simulink model "model"  (Simulink 7.9)
settings: Solver=ode3  StartTime=0.0  StopTime=5  FixedStep=0.001  RelTol=1e-3
values from neighbouring files (symbols this model uses):
  a = -1.0    (= -1)    [parameters.m]
  Ah = 0.234    [parameters.m]
  Ak = 0.227    [parameters.m]
  b = -2.0    (= -2)    [parameters.m]
  c = 0.23    [parameters.m]
  p = 0.1786    [parameters.m]
  Ta = 0.38    [parameters.m]
  Tr = 0.04    [parameters.m]
  U0 = 0.1*rand(4,4)    [parameters.m]
  W = [0 -1 1 -1; -1 0 -1 1; 1 -1 0 -1; -1 1 -1 0]    [parameters.m]
settings Model: Creator=dede  LastModifiedBy=dede

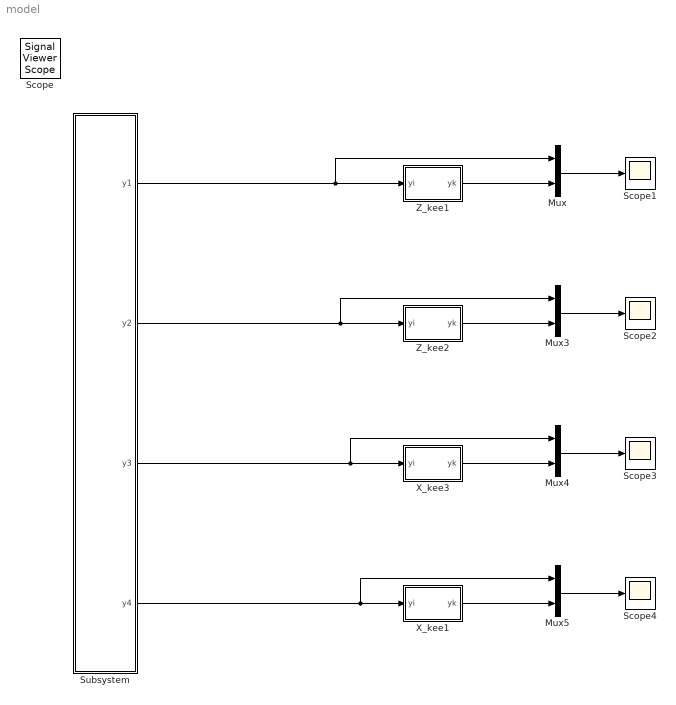
== system model ==
  Mux{,3..5} (4 alike) : Mux  Inputs=2
  Scope{1..4} (4 alike) : Scope
      Scope3 settings: SaveName=ScopeData2
      Scope4 settings: SaveName=ScopeData3
  Subsystem : Subsystem
  X_kee1 : Subsystem
  X_kee3 : Subsystem
  Z_kee1 : Subsystem
  Z_kee2 : Subsystem
  Scope : SignalViewerScope  IOType=viewer  NumInputPorts=4  RefreshTime=0.035000
      settings: YMin=-5~-5~-5~-5  YMax=5~5~5~5
  wires:
  Z_kee1/1(yk) -> Mux/2
  Mux/1 -> Scope1/1
  Z_kee2/1(yk) -> Mux3/2
  Mux3/1 -> Scope2/1
  X_kee3/1(yk) -> Mux4/2
  Mux4/1 -> Scope3/1
  Mux5/1 -> Scope4/1
  X_kee1/1(yk) -> Mux5/2
  Subsystem/4(y4) -> X_kee1/1(yi), Mux5/1
  Subsystem/3(y3) -> X_kee3/1(yi), Mux4/1
  Subsystem/2(y2) -> Z_kee2/1(yi), Mux3/1
  Subsystem/1(y1) -> Z_kee1/1(yi), Mux/1

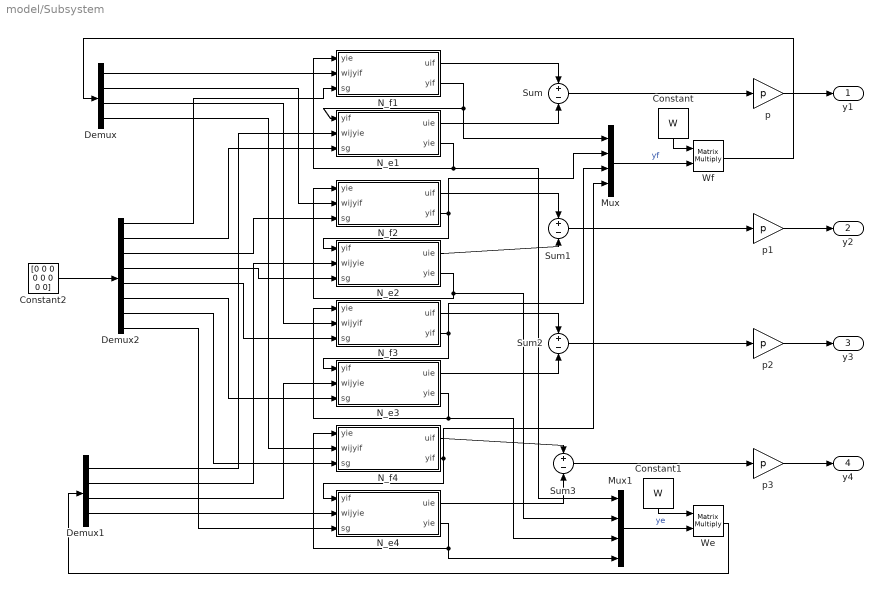
== system model/Subsystem ==
  Constant : Constant  Value=W
  Constant1 : Constant  Value=W
  Constant2 : Constant  Value=[0 0 0 0 0 0 0 0]
  Demux : Demux
  Demux1 : Demux
  Demux2 : Demux  Outputs=8
  Mux : Mux
  Mux1 : Mux
  N_e1 : Subsystem
  N_e2 : Subsystem
  N_e3 : Subsystem
  N_e4 : Subsystem
  N_f1 : Subsystem
  N_f2 : Subsystem
  N_f3 : Subsystem
  N_f4 : Subsystem
  Sum{,1..3} (4 alike) : Sum  Inputs=+-
  We : Product  Multiplication=Matrix(*)  RndMeth=Zero
  Wf : Product  Multiplication=Matrix(*)  RndMeth=Zero
  p{,1..3} (4 alike) : Gain  Gain=p
  y1 : Outport
  y2 : Outport  Port=2
  y3 : Outport  Port=3
  y4 : Outport  Port=4
  wires:
  N_f1/2(yif) -> N_e1/1(yif), Mux/1
  N_e1/2(yie) -> N_f1/1(yie), Mux1/1
  N_f2/2(yif) -> N_e2/1(yif), Mux/2
  N_e2/2(yie) -> N_f2/1(yie), Mux1/2
  N_f3/2(yif) -> N_e3/1(yif), Mux/3
  N_e3/2(yie) -> N_f3/1(yie), Mux1/3
  N_f4/2(yif) -> N_e4/1(yif), Mux/4
  N_e4/2(yie) -> N_f4/1(yie), Mux1/4
  N_f1/1(uif) -> Sum/1
  N_e1/1(uie) -> Sum/2
  N_f2/1(uif) -> Sum1/1
  N_e2/1(uie) -> Sum1/2
  N_f3/1(uif) -> Sum2/1
  N_e3/1(uie) -> Sum2/2
  N_f4/1(uif) -> Sum3/1
  N_e4/1(uie) -> Sum3/2
  Sum/1 -> p/1
  Mux/1 -> Wf/2  "yf"
  Constant/1 -> Wf/1
  Wf/1 -> Demux/1
  Mux1/1 -> We/2  "ye"
  Constant1/1 -> We/1
  We/1 -> Demux1/1
  Demux/1 -> N_f1/2(wijyif)
  Demux/2 -> N_f2/2(wijyif)
  Demux/3 -> N_f3/2(wijyif)
  Demux/4 -> N_f4/2(wijyif)
  Demux1/1 -> N_e1/2(wijyie)
  Demux1/2 -> N_e2/2(wijyie)
  Demux1/3 -> N_e3/2(wijyie)
  Demux1/4 -> N_e4/2(wijyie)
  Constant2/1 -> Demux2/1
  Demux2/1 -> N_f1/3(sg)
  Demux2/2 -> N_e1/3(sg)
  Demux2/3 -> N_f2/3(sg)
  Demux2/4 -> N_e2/3(sg)
  Demux2/5 -> N_f3/3(sg)
  Demux2/6 -> N_e3/3(sg)
  Demux2/7 -> N_f4/3(sg)
  Demux2/8 -> N_e4/3(sg)
  Sum1/1 -> p1/1
  p1/1 -> y2/1
  Sum2/1 -> p2/1
  p2/1 -> y3/1
  Sum3/1 -> p3/1
  p3/1 -> y4/1
  p/1 -> y1/1

== system model/X_kee1 ==
  yi : Inport
  Constant2 : Constant  Value=0
  Derivative : Derivative
  Subsystem : Subsystem
  Switch : Switch
  yk : Outport
  wires:
  Switch/1 -> yk/1
  Subsystem/1(Out1) -> Switch/1
  Derivative/1 -> Switch/2
  yi/1 -> Subsystem/1(In1), Derivative/1
  Constant2/1 -> Switch/3

== system model/X_kee3 ==
  yi : Inport
  Constant2 : Constant  Value=0
  Derivative : Derivative
  Subsystem : Subsystem
  Switch : Switch
  yk : Outport
  wires:
  Constant2/1 -> Switch/3
  yi/1 -> Derivative/1, Subsystem/1(In1)
  Derivative/1 -> Switch/2
  Subsystem/1(Out1) -> Switch/1
  Switch/1 -> yk/1

== system model/Z_kee1 ==
  yi : Inport
  Constant2 : Constant  Value=0
  Derivative : Derivative
  Subsystem : Subsystem
  Switch : Switch
  yk : Outport
  wires:
  Constant2/1 -> Switch/3
  yi/1 -> Derivative/1, Subsystem/1(In1)
  Derivative/1 -> Switch/2
  Subsystem/1(Out1) -> Switch/1
  Switch/1 -> yk/1

== system model/Z_kee2 ==
  yi : Inport
  Constant2 : Constant  Value=0
  Derivative : Derivative
  Subsystem : Subsystem
  Switch : Switch
  yk : Outport
  wires:
  Switch/1 -> yk/1
  Subsystem/1(Out1) -> Switch/1
  Derivative/1 -> Switch/2
  yi/1 -> Subsystem/1(In1), Derivative/1
  Constant2/1 -> Switch/3

== system model/Subsystem/N_e1 ==
  yif : Inport
  wijyie : Inport  Port=2
  sg : Inport  Port=3
  Constant : Constant  Value=0
  uie0 : Subsystem
  vie : Subsystem
  yie0 : Switch
  uie : Outport
  yie : Outport  Port=2
  wires:
  vie/1(vie) -> uie0/1(vie)
  yif/1 -> uie0/2(yif)
  wijyie/1 -> uie0/3(wijyie)
  Constant/1 -> yie0/3
  uie0/1(uie) -> yie0/1, yie0/2, uie/1
  yie0/1 -> vie/1(yie), yie/1
  sg/1 -> uie0/4(sg)

== system model/Subsystem/N_e2 ==
  yif : Inport
  wijyie : Inport  Port=2
  sg : Inport  Port=3
  Constant : Constant  Value=0
  uie0 : Subsystem
  vie : Subsystem
  yie0 : Switch
  uie : Outport
  yie : Outport  Port=2
  wires:
  sg/1 -> uie0/4(sg)
  yie0/1 -> yie/1, vie/1(yie)
  uie0/1(uie) -> uie/1, yie0/2, yie0/1
  Constant/1 -> yie0/3
  wijyie/1 -> uie0/3(wijyie)
  yif/1 -> uie0/2(yif)
  vie/1(vie) -> uie0/1(vie)

== system model/Subsystem/N_e3 ==
  yif : Inport
  wijyie : Inport  Port=2
  sg : Inport  Port=3
  Constant : Constant  Value=0
  uie0 : Subsystem
  vie : Subsystem
  yie0 : Switch
  uie : Outport
  yie : Outport  Port=2
  wires:
  vie/1(vie) -> uie0/1(vie)
  yif/1 -> uie0/2(yif)
  wijyie/1 -> uie0/3(wijyie)
  Constant/1 -> yie0/3
  uie0/1(uie) -> yie0/1, yie0/2, uie/1
  yie0/1 -> vie/1(yie), yie/1
  sg/1 -> uie0/4(sg)

== system model/Subsystem/N_e4 ==
  yif : Inport
  wijyie : Inport  Port=2
  sg : Inport  Port=3
  Constant : Constant  Value=0
  uie0 : Subsystem
  vie : Subsystem
  yie0 : Switch
  uie : Outport
  yie : Outport  Port=2
  wires:
  sg/1 -> uie0/4(sg)
  yie0/1 -> yie/1, vie/1(yie)
  uie0/1(uie) -> uie/1, yie0/2, yie0/1
  Constant/1 -> yie0/3
  wijyie/1 -> uie0/3(wijyie)
  yif/1 -> uie0/2(yif)
  vie/1(vie) -> uie0/1(vie)

== system model/Subsystem/N_f1 ==
  yie : Inport
  wijyif : Inport  Port=2
  sg : Inport  Port=3
  Constant : Constant  Value=0
  uif0 : Subsystem
  vif : Subsystem
  yif0 : Switch
  uif : Outport
  yif : Outport  Port=2
  wires:
  vif/1(vif) -> uif0/1(vif)
  Constant/1 -> yif0/3
  uif0/1(uif) -> yif0/1, yif0/2, uif/1
  yif0/1 -> yif/1, vif/1(yif)
  yie/1 -> uif0/2(yie)
  wijyif/1 -> uif0/3(wijyif)
  sg/1 -> uif0/4(sg)

== system model/Subsystem/N_f2 ==
  yie : Inport
  wijyif : Inport  Port=2
  sg : Inport  Port=3
  Constant : Constant  Value=0
  uif0 : Subsystem
  vif : Subsystem
  yif0 : Switch
  uif : Outport
  yif : Outport  Port=2
  wires:
  sg/1 -> uif0/4(sg)
  wijyif/1 -> uif0/3(wijyif)
  yie/1 -> uif0/2(yie)
  yif0/1 -> yif/1, vif/1(yif1)
  uif0/1(uif) -> uif/1, yif0/2, yif0/1
  Constant/1 -> yif0/3
  vif/1(vif) -> uif0/1(vif)

== system model/Subsystem/N_f3 ==
  yie : Inport
  wijyif : Inport  Port=2
  sg : Inport  Port=3
  Constant : Constant  Value=0
  uif0 : Subsystem
  vif : Subsystem
  yif0 : Switch
  uif : Outport
  yif : Outport  Port=2
  wires:
  vif/1(vif) -> uif0/1(vif)
  Constant/1 -> yif0/3
  uif0/1(uif) -> yif0/1, yif0/2, uif/1
  yif0/1 -> vif/1(yif1), yif/1
  yie/1 -> uif0/2(yie)
  wijyif/1 -> uif0/3(wijyif)
  sg/1 -> uif0/4(sg)

== system model/Subsystem/N_f4 ==
  yie : Inport
  wijyif : Inport  Port=2
  sg : Inport  Port=3
  Constant : Constant  Value=0
  uif0 : Subsystem
  vif : Subsystem
  yif0 : Switch
  uif : Outport
  yif : Outport  Port=2
  wires:
  sg/1 -> uif0/4(sg)
  wijyif/1 -> uif0/3(wijyif)
  yie/1 -> uif0/2(yie)
  yif0/1 -> yif/1, vif/1(yif1)
  uif0/1(uif) -> uif/1, yif0/2, yif0/1
  Constant/1 -> yif0/3
  vif/1(vif) -> uif0/1(vif)

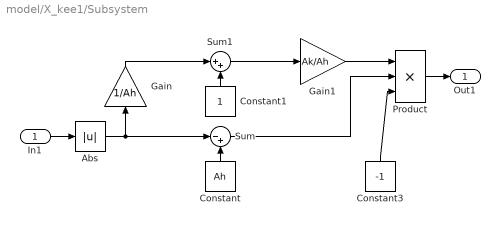
== system model/X_kee1/Subsystem ==
  In1 : Inport
  Abs : Abs
  Constant : Constant  Value=Ah
  Constant1 : Constant
  Constant3 : Constant  Value=-1
  Gain : Gain  Gain=1/Ah
  Gain1 : Gain  Gain=Ak/Ah
  Product : Product  Inputs=3  RndMeth=Zero
  Sum : Sum  Inputs=|-+
  Sum1 : Sum  Inputs=|++
  Out1 : Outport
  wires:
  In1/1 -> Abs/1
  Product/1 -> Out1/1
  Constant3/1 -> Product/3
  Gain1/1 -> Product/1
  Sum/1 -> Product/2
  Sum1/1 -> Gain1/1
  Gain/1 -> Sum1/1
  Constant1/1 -> Sum1/2
  Constant/1 -> Sum/2
  Abs/1 -> Gain/1, Sum/1

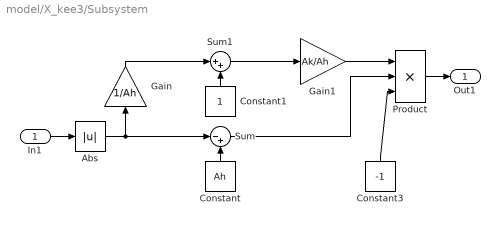
== system model/X_kee3/Subsystem ==
  In1 : Inport
  Abs : Abs
  Constant : Constant  Value=Ah
  Constant1 : Constant
  Constant3 : Constant  Value=-1
  Gain : Gain  Gain=1/Ah
  Gain1 : Gain  Gain=Ak/Ah
  Product : Product  Inputs=3  RndMeth=Zero
  Sum : Sum  Inputs=|-+
  Sum1 : Sum  Inputs=|++
  Out1 : Outport
  wires:
  Abs/1 -> Sum/1, Gain/1
  Constant/1 -> Sum/2
  Constant1/1 -> Sum1/2
  Gain/1 -> Sum1/1
  Sum1/1 -> Gain1/1
  Sum/1 -> Product/2
  Gain1/1 -> Product/1
  Constant3/1 -> Product/3
  Product/1 -> Out1/1
  In1/1 -> Abs/1

== system model/Z_kee1/Subsystem ==
  In1 : Inport
  Abs : Abs
  Constant : Constant  Value=Ah
  Constant1 : Constant
  Gain : Gain  Gain=1/Ah
  Gain1 : Gain  Gain=Ak/Ah
  Product : Product  RndMeth=Zero
  Sum : Sum  Inputs=|-+
  Sum1 : Sum  Inputs=|++
  Out1 : Outport
  wires:
  Abs/1 -> Sum/1, Gain/1
  Constant/1 -> Sum/2
  Constant1/1 -> Sum1/2
  Gain/1 -> Sum1/1
  Sum1/1 -> Gain1/1
  Sum/1 -> Product/2
  Gain1/1 -> Product/1
  Product/1 -> Out1/1
  In1/1 -> Abs/1

== system model/Z_kee2/Subsystem ==
  In1 : Inport
  Abs : Abs
  Constant : Constant  Value=Ah
  Constant1 : Constant
  Gain : Gain  Gain=1/Ah
  Gain1 : Gain  Gain=Ak/Ah
  Product : Product  RndMeth=Zero
  Sum : Sum  Inputs=|-+
  Sum1 : Sum  Inputs=|++
  Out1 : Outport
  wires:
  In1/1 -> Abs/1
  Product/1 -> Out1/1
  Gain1/1 -> Product/1
  Sum/1 -> Product/2
  Sum1/1 -> Gain1/1
  Gain/1 -> Sum1/1
  Constant1/1 -> Sum1/2
  Constant/1 -> Sum/2
  Abs/1 -> Gain/1, Sum/1

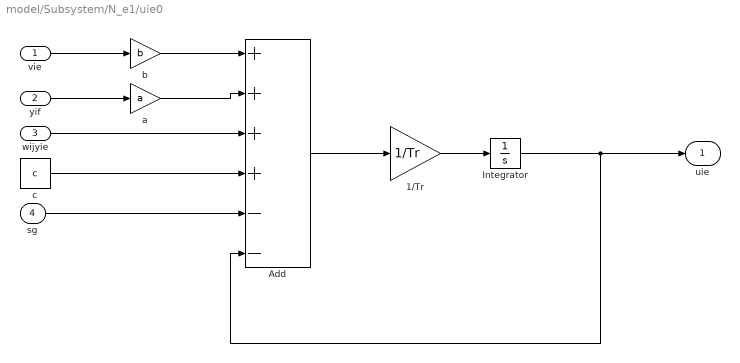
== system model/Subsystem/N_e1/uie0 ==
  vie : Inport
  yif : Inport  Port=2
  wijyie : Inport  Port=3
  sg : Inport  Port=4
  1/Tr : Gain  Gain=1/Tr
  Add : Sum  Inputs=++++--
  Integrator : Integrator  InitialCondition=U0(3,1)
  a : Gain  Gain=a
  b : Gain  Gain=b
  c : Constant  Value=c
  uie : Outport
  wires:
  vie/1 -> b/1
  b/1 -> Add/1
  yif/1 -> a/1
  a/1 -> Add/2
  wijyie/1 -> Add/3
  c/1 -> Add/4
  Add/1 -> 1/Tr/1
  1/Tr/1 -> Integrator/1
  Integrator/1 -> uie/1, Add/6
  sg/1 -> Add/5

== system model/Subsystem/N_e1/vie ==
  yie : Inport
  1/Ta : Gain  Gain=1/Ta
  1/Ta1 : Gain  Gain=1/Ta
  Add : Sum  Inputs=+-
  Integrator : Integrator  InitialCondition=U0(4,1)
  vie : Outport
  wires:
  yie/1 -> 1/Ta/1
  1/Ta/1 -> Add/1
  Add/1 -> Integrator/1
  Integrator/1 -> 1/Ta1/1, vie/1
  1/Ta1/1 -> Add/2

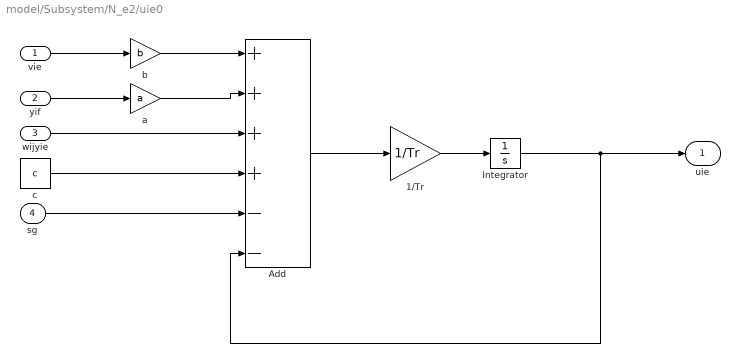
== system model/Subsystem/N_e2/uie0 ==
  vie : Inport
  yif : Inport  Port=2
  wijyie : Inport  Port=3
  sg : Inport  Port=4
  1/Tr : Gain  Gain=1/Tr
  Add : Sum  Inputs=++++--
  Integrator : Integrator  InitialCondition=U0(3,2)
  a : Gain  Gain=a
  b : Gain  Gain=b
  c : Constant  Value=c
  uie : Outport
  wires:
  sg/1 -> Add/5
  Integrator/1 -> Add/6, uie/1
  1/Tr/1 -> Integrator/1
  Add/1 -> 1/Tr/1
  c/1 -> Add/4
  wijyie/1 -> Add/3
  a/1 -> Add/2
  yif/1 -> a/1
  b/1 -> Add/1
  vie/1 -> b/1

== system model/Subsystem/N_e2/vie ==
  yie : Inport
  1/Ta : Gain  Gain=1/Ta
  1/Ta1 : Gain  Gain=1/Ta
  Add : Sum  Inputs=+-
  Integrator : Integrator  InitialCondition=U0(4,2)
  vie : Outport
  wires:
  1/Ta1/1 -> Add/2
  Integrator/1 -> vie/1, 1/Ta1/1
  Add/1 -> Integrator/1
  1/Ta/1 -> Add/1
  yie/1 -> 1/Ta/1

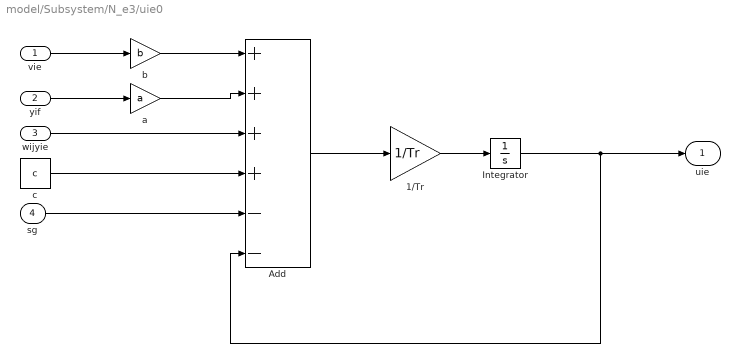
== system model/Subsystem/N_e3/uie0 ==
  vie : Inport
  yif : Inport  Port=2
  wijyie : Inport  Port=3
  sg : Inport  Port=4
  1/Tr : Gain  Gain=1/Tr
  Add : Sum  Inputs=++++--
  Integrator : Integrator  InitialCondition=U0(3,3)
  a : Gain  Gain=a
  b : Gain  Gain=b
  c : Constant  Value=c
  uie : Outport
  wires:
  vie/1 -> b/1
  b/1 -> Add/1
  yif/1 -> a/1
  a/1 -> Add/2
  wijyie/1 -> Add/3
  c/1 -> Add/4
  Add/1 -> 1/Tr/1
  1/Tr/1 -> Integrator/1
  Integrator/1 -> uie/1, Add/6
  sg/1 -> Add/5

== system model/Subsystem/N_e3/vie ==
  yie : Inport
  1/Ta : Gain  Gain=1/Ta
  1/Ta1 : Gain  Gain=1/Ta
  Add : Sum  Inputs=+-
  Integrator : Integrator  InitialCondition=U0(4,3)
  vie : Outport
  wires:
  yie/1 -> 1/Ta/1
  1/Ta/1 -> Add/1
  Add/1 -> Integrator/1
  Integrator/1 -> 1/Ta1/1, vie/1
  1/Ta1/1 -> Add/2

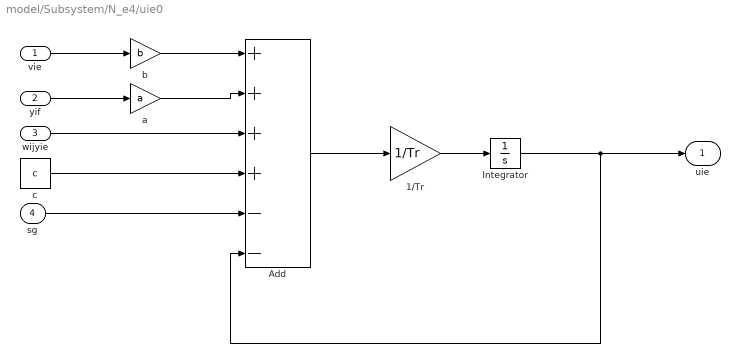
== system model/Subsystem/N_e4/uie0 ==
  vie : Inport
  yif : Inport  Port=2
  wijyie : Inport  Port=3
  sg : Inport  Port=4
  1/Tr : Gain  Gain=1/Tr
  Add : Sum  Inputs=++++--
  Integrator : Integrator  InitialCondition=U0(3,4)
  a : Gain  Gain=a
  b : Gain  Gain=b
  c : Constant  Value=c
  uie : Outport
  wires:
  sg/1 -> Add/5
  Integrator/1 -> Add/6, uie/1
  1/Tr/1 -> Integrator/1
  Add/1 -> 1/Tr/1
  c/1 -> Add/4
  wijyie/1 -> Add/3
  a/1 -> Add/2
  yif/1 -> a/1
  b/1 -> Add/1
  vie/1 -> b/1

== system model/Subsystem/N_e4/vie ==
  yie : Inport
  1/Ta : Gain  Gain=1/Ta
  1/Ta1 : Gain  Gain=1/Ta
  Add : Sum  Inputs=+-
  Integrator : Integrator  InitialCondition=U0(4,4)
  vie : Outport
  wires:
  1/Ta1/1 -> Add/2
  Integrator/1 -> vie/1, 1/Ta1/1
  Add/1 -> Integrator/1
  1/Ta/1 -> Add/1
  yie/1 -> 1/Ta/1

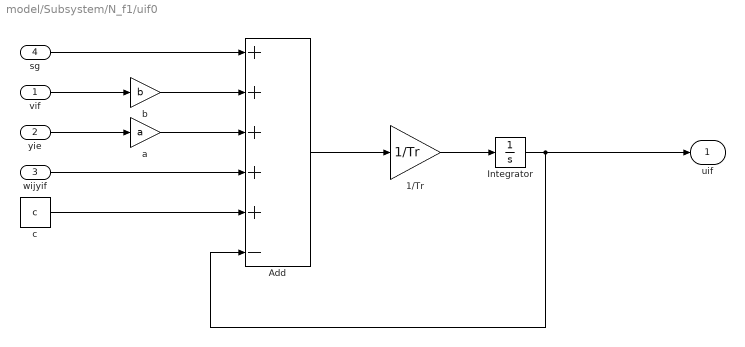
== system model/Subsystem/N_f1/uif0 ==
  vif : Inport
  yie : Inport  Port=2
  wijyif : Inport  Port=3
  sg : Inport  Port=4
  1/Tr : Gain  Gain=1/Tr
  Add : Sum  Inputs=+++++-
  Integrator : Integrator  InitialCondition=U0(1,1)
  a : Gain  Gain=a
  b : Gain  Gain=b
  c : Constant  Value=c
  uif : Outport
  wires:
  vif/1 -> b/1
  yie/1 -> a/1
  Add/1 -> 1/Tr/1
  1/Tr/1 -> Integrator/1
  Integrator/1 -> uif/1, Add/6
  b/1 -> Add/2
  a/1 -> Add/3
  wijyif/1 -> Add/4
  c/1 -> Add/5
  sg/1 -> Add/1

== system model/Subsystem/N_f1/vif ==
  yif : Inport
  1/Ta : Gain  Gain=1/Ta
  1/Ta1 : Gain  Gain=1/Ta
  Add : Sum  Inputs=+-
  Integrator : Integrator  InitialCondition=U0(2,1)
  vif : Outport
  wires:
  yif/1 -> 1/Ta/1
  1/Ta/1 -> Add/1
  Add/1 -> Integrator/1
  Integrator/1 -> 1/Ta1/1, vif/1
  1/Ta1/1 -> Add/2

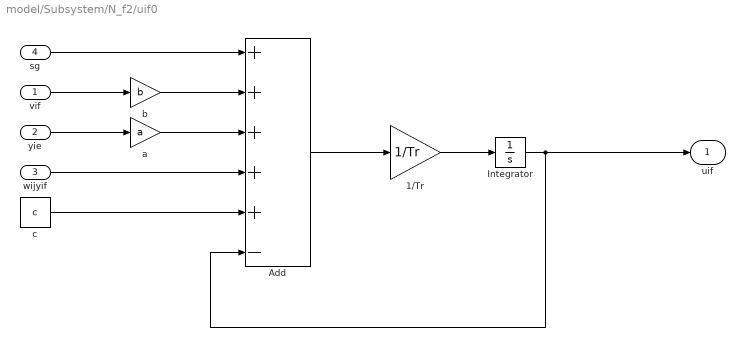
== system model/Subsystem/N_f2/uif0 ==
  vif : Inport
  yie : Inport  Port=2
  wijyif : Inport  Port=3
  sg : Inport  Port=4
  1/Tr : Gain  Gain=1/Tr
  Add : Sum  Inputs=+++++-
  Integrator : Integrator  InitialCondition=U0(1,2)
  a : Gain  Gain=a
  b : Gain  Gain=b
  c : Constant  Value=c
  uif : Outport
  wires:
  sg/1 -> Add/1
  c/1 -> Add/5
  wijyif/1 -> Add/4
  a/1 -> Add/3
  b/1 -> Add/2
  Integrator/1 -> Add/6, uif/1
  1/Tr/1 -> Integrator/1
  Add/1 -> 1/Tr/1
  yie/1 -> a/1
  vif/1 -> b/1

== system model/Subsystem/N_f2/vif ==
  yif1 : Inport
  1/Ta : Gain  Gain=1/Ta
  1/Ta1 : Gain  Gain=1/Ta
  Add : Sum  Inputs=+-
  Integrator : Integrator  InitialCondition=U0(2,2)
  vif : Outport
  wires:
  1/Ta1/1 -> Add/2
  Integrator/1 -> vif/1, 1/Ta1/1
  Add/1 -> Integrator/1
  1/Ta/1 -> Add/1
  yif1/1 -> 1/Ta/1

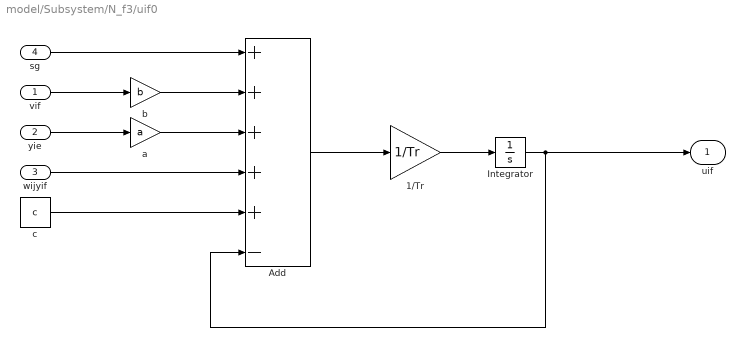
== system model/Subsystem/N_f3/uif0 ==
  vif : Inport
  yie : Inport  Port=2
  wijyif : Inport  Port=3
  sg : Inport  Port=4
  1/Tr : Gain  Gain=1/Tr
  Add : Sum  Inputs=+++++-
  Integrator : Integrator  InitialCondition=U0(3,1)
  a : Gain  Gain=a
  b : Gain  Gain=b
  c : Constant  Value=c
  uif : Outport
  wires:
  vif/1 -> b/1
  yie/1 -> a/1
  Add/1 -> 1/Tr/1
  1/Tr/1 -> Integrator/1
  Integrator/1 -> uif/1, Add/6
  b/1 -> Add/2
  a/1 -> Add/3
  wijyif/1 -> Add/4
  c/1 -> Add/5
  sg/1 -> Add/1

== system model/Subsystem/N_f3/vif ==
  yif1 : Inport
  1/Ta : Gain  Gain=1/Ta
  1/Ta1 : Gain  Gain=1/Ta
  Add : Sum  Inputs=+-
  Integrator : Integrator  InitialCondition=U0(3,2)
  vif : Outport
  wires:
  yif1/1 -> 1/Ta/1
  1/Ta/1 -> Add/1
  Add/1 -> Integrator/1
  Integrator/1 -> 1/Ta1/1, vif/1
  1/Ta1/1 -> Add/2

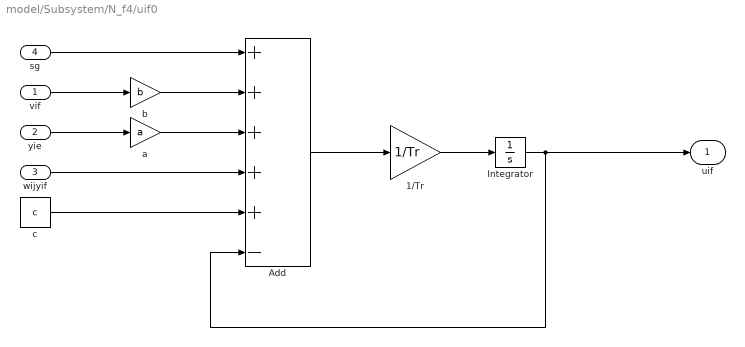
== system model/Subsystem/N_f4/uif0 ==
  vif : Inport
  yie : Inport  Port=2
  wijyif : Inport  Port=3
  sg : Inport  Port=4
  1/Tr : Gain  Gain=1/Tr
  Add : Sum  Inputs=+++++-
  Integrator : Integrator  InitialCondition=U0(1,4)
  a : Gain  Gain=a
  b : Gain  Gain=b
  c : Constant  Value=c
  uif : Outport
  wires:
  sg/1 -> Add/1
  c/1 -> Add/5
  wijyif/1 -> Add/4
  a/1 -> Add/3
  b/1 -> Add/2
  Integrator/1 -> Add/6, uif/1
  1/Tr/1 -> Integrator/1
  Add/1 -> 1/Tr/1
  yie/1 -> a/1
  vif/1 -> b/1

== system model/Subsystem/N_f4/vif ==
  yif1 : Inport
  1/Ta : Gain  Gain=1/Ta
  1/Ta1 : Gain  Gain=1/Ta
  Add : Sum  Inputs=+-
  Integrator : Integrator  InitialCondition=U0(2,4)
  vif : Outport
  wires:
  1/Ta1/1 -> Add/2
  Integrator/1 -> vif/1, 1/Ta1/1
  Add/1 -> Integrator/1
  1/Ta/1 -> Add/1
  yif1/1 -> 1/Ta/1
